simulink model "Complmentary3"  (R2021a)
settings: Solver=FixedStepAuto  StartTime=0.0  StopTime=Inf  RelTol=1e-3  EnableMultiTasking=on
libraries: arduinosensorlib x1
settings Model: SILPILModeSetting=veronly  ExtModeTrigDuration=2  Creator=user  LastModifiedBy=user
settings OptimizationCC: EnhancedBackFolding=on  PassReuseOutputArgsAs=Individual arguments  ZeroExternalMemoryAtStartup=off  ZeroInternalMemoryAtStartup=off  MaxStackSize=64  OptimizeBlockOrder=speed  DifferentSizesBufferReuse=on  OptimizationCustomize=off  EfficientTunableParamExpr=on
settings DebuggingCC: ParameterTunabilityLossMsg=error
settings HardwareCC: ProdBitPerInt=16  ProdBitPerPointer=16  ProdBitPerSizeT=16  ProdBitPerPtrDiffT=16  ProdLargestAtomicFloat=None  ProdWordSize=8  ProdHWDeviceType=Atmel->AVR  UseEmbeddedCoderFeatures=off  UseSimulinkCoderFeatures=off
settings SFSimCC: MATLABDynamicMemAlloc=off
settings RTWCC: SystemTargetFile=ert.tlc  HardwareBoard=Arduino Uno  TemplateMakefile=ert_default_tmf  Toolchain=Arduino AVR  BuildConfiguration=Faster Runs
settings CodeAppCC: ForceParamTrailComments=on  IgnoreCustomStorageClasses=off  OperatorAnnotations=on  SimulinkDataObjDesc=on  SFDataObjDesc=on  InsertBlockDesc=on
settings ERTTargetCC: SupportContinuousTime=on  SupportNonInlinedSFcns=on  SupportVariableSizeSignals=on  ExtModeStaticAllocSize=250

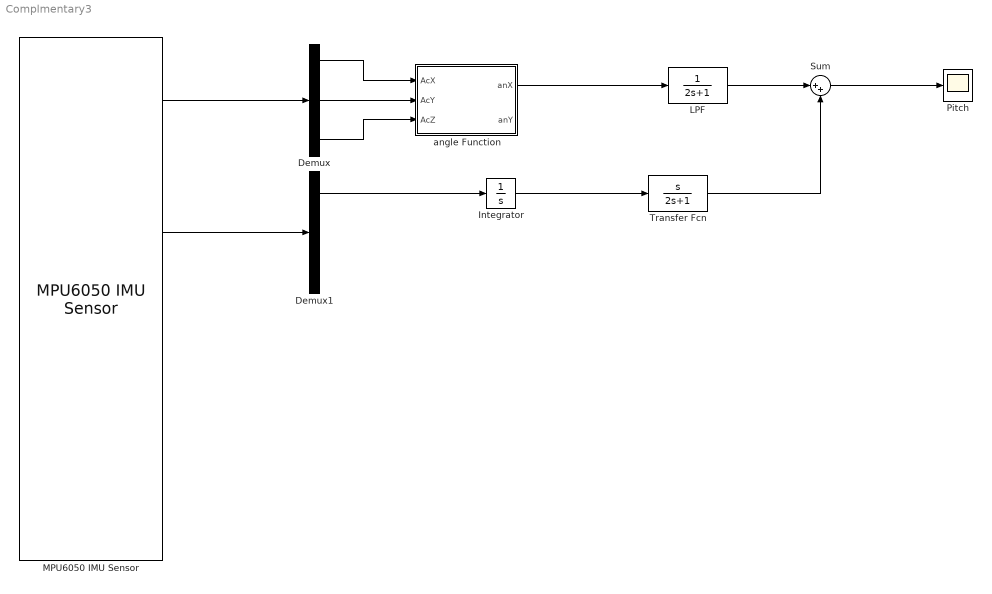
== system Complmentary3 ==
  Demux : Demux  Outputs=3
  Demux1 : Demux  Outputs=3
  Integrator : Integrator
  LPF : TransferFcn  Denominator=[2 1]
  MPU6050 IMU Sensor : arduinosensorlib/MPU6050 IMU Sensor  SlaveAddress=0x68  Accel=on  AngularRate=on  Temperature=on  Status=on  EulerAngles=off  Quat=off  AccelRange=2G  GyroRange=250 dps  DmpOdr=200 Hz  Dlpf=Accelerometer: 184Hz, Gyroscope: 188Hz  SampleTime=-1
      settings: SourceProductBaseCode=ARDUINO
  Pitch : Scope
  Sum : Sum  Inputs=|++
  Transfer Fcn : TransferFcn  Numerator=[1 0]  Denominator=[2 1]
  angle Function : MATLAB Function  TreatAsAtomicUnit=on
  wires:
  MPU6050 IMU Sensor/1 -> Demux/1
  Demux/1 -> angle Function/1(AcX)
  Demux/2 -> angle Function/2(AcY)
  Demux/3 -> angle Function/3(AcZ)
  angle Function/1(anX) -> LPF/1
  MPU6050 IMU Sensor/2 -> Demux1/1
  LPF/1 -> Sum/1
  Demux1/1 -> Integrator/1
  Integrator/1 -> Transfer Fcn/1
  Transfer Fcn/1 -> Sum/2
  Sum/1 -> Pitch/1

== matlab function Complmentary3/angle Function ==
  data: AcX input; anX output; AcY input; AcZ input; anY output
function [anX,anY] = fcn(AcX,AcY,AcZ)

anX = atan(-AcY / (sqrt(AcX^2 + AcZ^2))) * 180/pi;
anY = atan(-AcX / (sqrt(AcY^2 + AcZ^2))) * 180/pi;

end
